simulink model "zadM3a"  (R2021b)
settings: Solver=VariableStepAuto  StartTime=0.0  StopTime=10.0  RelTol=1e-3
settings Model: Creator=Studenci  LastModifiedBy=Studenci

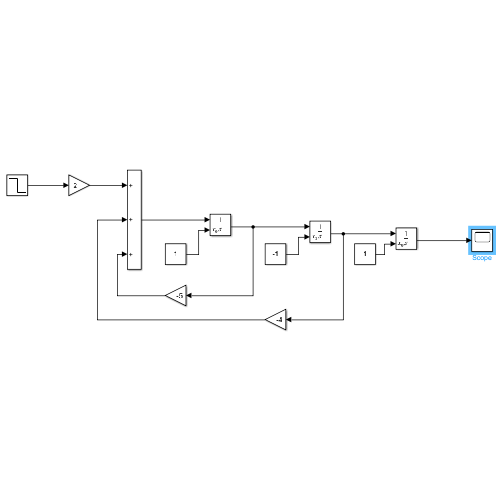
[thumbnail: Simulink's stored preview of the top-level diagram]
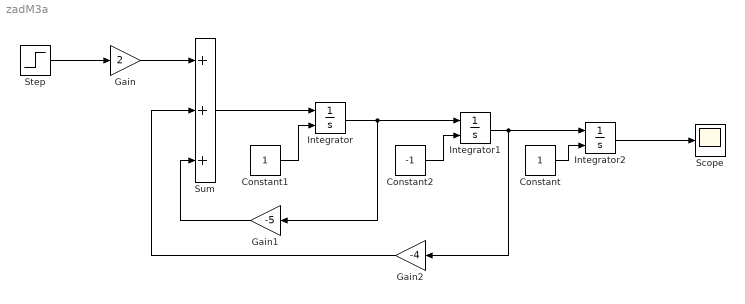
== system zadM3a ==
  Constant : Constant
  Constant1 : Constant
  Constant2 : Constant  Value=-1
  Gain : Gain  Gain=2
  Gain1 : Gain  Gain=-5
  Gain2 : Gain  Gain=-4
  Integrator : Integrator  InitialConditionSource=external
  Integrator1 : Integrator  InitialConditionSource=external
  Integrator2 : Integrator  InitialConditionSource=external
  Scope : Scope
  Step : Step  Time=0.01  Before=100  After=0  SampleTime=0
  Sum : Sum  Inputs=+++
  wires:
  Constant1/1 -> Integrator/2
  Constant2/1 -> Integrator1/2
  Constant/1 -> Integrator2/2
  Step/1 -> Gain/1
  Gain/1 -> Sum/1
  Sum/1 -> Integrator/1
  Integrator/1 -> Gain1/1, Integrator1/1
  Integrator1/1 -> Gain2/1, Integrator2/1
  Gain1/1 -> Sum/3
  Gain2/1 -> Sum/2
  Integrator2/1 -> Scope/1
